simulink model "sampleModel1434"  (R2023a)
settings: Solver=VariableStepAuto  StartTime=0.0  StopTime=10.0  RelTol=1e-3
libraries: hdlsllib x3, simulink x1
settings Model: Creator=user1  LastModifiedBy=user1

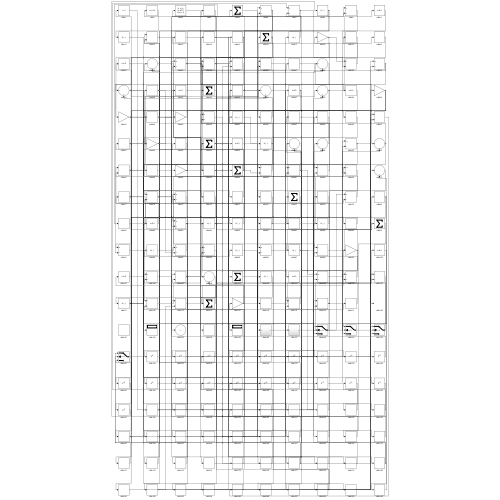
[thumbnail: Simulink's stored preview of the top-level diagram]
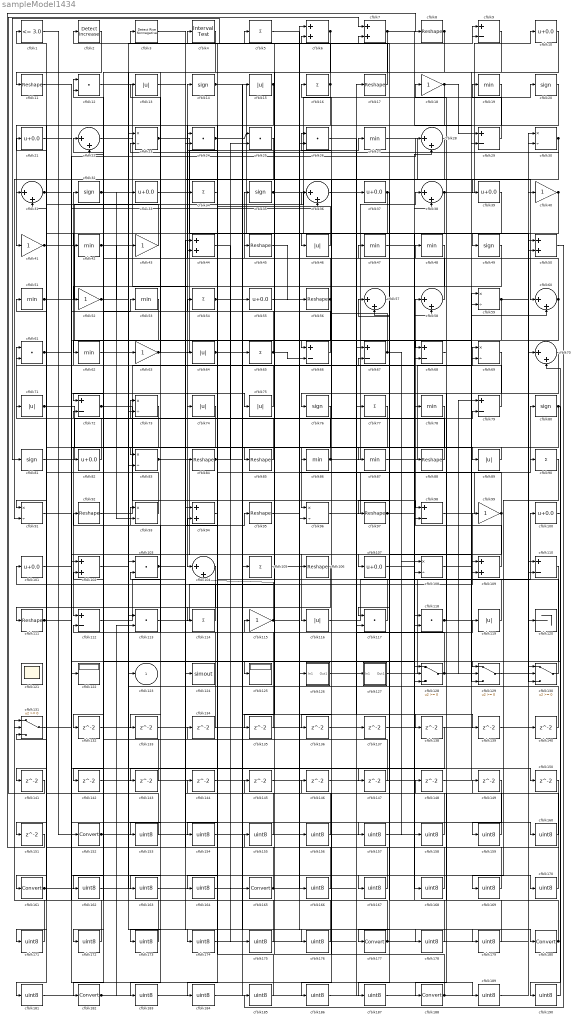
== system sampleModel1434 ==
  cfblk1 : hdlsllib/Logic and Bit Operations/Compare To Constant  relop=<=  const=3.0  OutDataTypeStr=boolean
  cfblk{10,21,33,37,39,55,82,100..101,107} (10 alike) : Bias  Bias=0.0  SaturateOnIntegerOverflow=off
  cfblk{6..7,44,50,94,102,109} (7 alike) : Sum
  cfblk{12,24..26,61,103,113,117..118} (9 alike) : DotProduct  OutDataTypeStr=Inherit: Inherit via internal rule
  cfblk{22,28,31,36,38,57..58,60,70,104} (10 alike) : Sum  Inputs=|++
  cfblk{5,16,34,54,65,77,90,105,114} (9 alike) : Sum  Inputs=+
  cfblk{8,11,17,45,56,84..85,88,92,95,97,106,111} (13 alike) : Reshape
  cfblk{23,30,59,69,73,83,91,93,96,108} (10 alike) : Product  Inputs=*/  RndMeth=Zero  SaturateOnIntegerOverflow=on
  cfblk{9,29,66..68,72,79,98,110,112} (10 alike) : Sum  Inputs=+-
  cfblk{18,40..41,43,52,63,99,115} (8 alike) : Gain
  cfblk{13,15,46,64,71,74..75,89,116,119} (10 alike) : Abs  SaturateOnIntegerOverflow=off
  cfblk120 : Terminator
  cfblk121 : Scope
      settings: Floating=on
  cfblk122 : Display
  cfblk124 : ToWorkspace  VariableName=simout  SaveFormat=Timeseries  SampleTime=-1
  cfblk125 : Display
  cfblk126 : Subsystem
      settings: LibrarySourceBlock=|
      | hdlsllib/Ports &
      | Subsystems/Subsystem
  cfblk127 : Subsystem
      settings: LibrarySourceBlock=|
      | hdlsllib/Ports &
      | Subsystems/Subsystem
  cfblk{128..131} (4 alike) : Switch  SaturateOnIntegerOverflow=off  InputSameDT=off
  cfblk{132..151} (20 alike) : Delay  SampleTime=1
  cfblk{14,20,32,35,49,76,80..81} (8 alike) : Signum
  cfblk{152,161,165,177,180,182,188} (7 alike) : DataTypeConversion  SaturateOnIntegerOverflow=off  RndMeth=Floor
  cfblk{153..160,162..164,166..176,178..179,181,183..187,189..190} (32 alike) : DataTypeConversion  OutDataTypeStr=uint8  SaturateOnIntegerOverflow=off  RndMeth=Floor
  cfblk{19,27,42,47..48,51,53,62,78,86..87} (11 alike) : MinMax
  cfblk2 : simulink/Logic and Bit Operations/Detect Increase  vinit=0.0  OutDataTypeStr=boolean
      settings: LibrarySourceBlock=|
      | hdlsllib/Logic and Bit
      | Operations/Detect
      | Increase
  cfblk3 : hdlsllib/Logic and Bit Operations/Detect Rise Nonnegative  vinit=0  OutDataTypeStr=boolean
  cfblk4 : hdlsllib/Logic and Bit Operations/Interval Test  IntervalClosedRight=on  uplimit=0.5  IntervalClosedLeft=on  lowlimit=-0.5  OutDataTypeStr=boolean
  cfblk123 : Outport  VectorParamsAs1DForOutWhenUnconnected=off
  wires:
  cfblk109/1 -> cfblk58/1
  cfblk74/1 -> cfblk112/1
  cfblk54/1 -> cfblk36/1, cfblk138/1, cfblk178/1
  cfblk86/1 -> cfblk38/1, cfblk31/2
  cfblk45/1 -> cfblk56/1
  cfblk27/1 -> cfblk60/1
  cfblk58/1 -> cfblk14/1
  cfblk117/1 -> cfblk3/1
  cfblk17/1 -> cfblk81/1
  cfblk46/1 -> cfblk4/1
  cfblk84/1 -> cfblk25/2, cfblk167/1, cfblk175/1
  cfblk33/1 -> cfblk104/1
  cfblk63/1 -> cfblk27/1, cfblk13/1
  cfblk127/1(Out1) -> cfblk100/1
  cfblk83/1 -> cfblk116/1, cfblk143/1
  cfblk103/1 -> cfblk68/2, cfblk176/1
  cfblk40/1 -> cfblk108/2, cfblk141/1, cfblk142/1
  cfblk100/1 -> cfblk129/1
  cfblk111/1 -> cfblk53/1, cfblk36/2, cfblk28/1
  cfblk79/1 -> cfblk32/1
  cfblk119/1 -> cfblk7/2
  cfblk129/1 -> cfblk130/2
  cfblk77/1 -> cfblk161/1
  cfblk44/1 -> cfblk165/1
  cfblk51/1 -> cfblk20/1, cfblk147/1
  cfblk37/1 -> cfblk76/1, cfblk97/1
  cfblk89/1 -> cfblk87/1
  cfblk78/1 -> cfblk111/1
  cfblk23/1 -> cfblk46/1, cfblk65/1
  cfblk66/1 -> cfblk22/1
  cfblk112/1 -> cfblk95/1
  cfblk118/1 -> cfblk129/2, cfblk18/1
  cfblk62/1 -> cfblk9/1
  cfblk16/1 -> cfblk41/1, cfblk2/1, cfblk31/1
  cfblk73/1 -> cfblk91/1
  cfblk88/1 -> cfblk26/1
  cfblk20/1 -> cfblk34/1
  cfblk68/1 -> cfblk48/1
  cfblk60/1 -> cfblk62/1, cfblk22/2
  cfblk72/1 -> cfblk98/1, cfblk79/2
  cfblk92/1 -> cfblk17/1
  cfblk14/1 -> cfblk49/1, cfblk128/3
  cfblk115/1 -> cfblk104/2, cfblk101/1, cfblk90/1
  cfblk56/1 -> cfblk35/1, cfblk83/2
  cfblk85/1 -> cfblk73/1
  cfblk38/1 -> cfblk10/1, cfblk173/1
  cfblk71/1 -> cfblk89/1, cfblk189/1
  cfblk87/1 -> cfblk69/1
  cfblk107/1 -> cfblk78/1
  cfblk70/1 -> cfblk188/1
  cfblk25/1 -> cfblk91/2
  cfblk128/1 -> cfblk59/2, cfblk79/1, cfblk12/2
  cfblk130/1 -> cfblk92/1
  cfblk6/1 -> cfblk85/1, cfblk183/1
  cfblk101/1 -> cfblk107/1
  cfblk59/1 -> cfblk130/3, cfblk118/2
  cfblk28/1 -> cfblk66/1
  cfblk29/1 -> cfblk19/1
  cfblk32/1 -> cfblk64/1, cfblk93/2
  cfblk30/1 -> cfblk23/2, cfblk132/1
  cfblk7/1 -> cfblk72/1, cfblk29/2
  cfblk12/1 -> cfblk84/1
  cfblk98/1 -> cfblk80/1
  cfblk10/1 -> cfblk129/3
  cfblk26/1 -> cfblk69/2
  cfblk8/1 -> cfblk24/2, cfblk162/1
  cfblk64/1 -> cfblk15/1, cfblk179/1
  cfblk41/1 -> cfblk126/1(In1), cfblk160/1
  cfblk80/1 -> cfblk96/1, cfblk190/1
  cfblk13/1 -> cfblk39/1
  cfblk42/1 -> cfblk123/1, cfblk6/2
  cfblk31/1 -> cfblk83/1, cfblk75/1
  cfblk2/1 -> cfblk11/1
  cfblk113/1 -> cfblk99/1
  cfblk105/1 -> cfblk180/1
  cfblk49/1 -> cfblk52/1
  cfblk110/1 -> cfblk182/1
  cfblk116/1 -> cfblk40/1
  cfblk82/1 -> cfblk61/1
  cfblk35/1 -> cfblk120/1, cfblk9/2
  cfblk114/1 -> cfblk93/1
  cfblk97/1 -> cfblk88/1, cfblk108/1
  cfblk34/1 -> cfblk114/1
  cfblk43/1 -> cfblk21/1
  cfblk19/1 -> cfblk42/1
  cfblk57/1 -> cfblk177/1
  cfblk93/1 -> cfblk71/1
  cfblk91/1 -> cfblk122/1
  cfblk3/1 -> cfblk86/1
  cfblk99/1 -> cfblk54/1, cfblk117/1, cfblk187/1
  cfblk22/1 -> cfblk124/1
  cfblk65/1 -> cfblk24/1, cfblk12/1, cfblk66/2
  cfblk52/1 -> cfblk128/2, cfblk43/1
  cfblk24/1 -> cfblk25/1, cfblk109/2
  cfblk4/1 -> cfblk73/2
  cfblk75/1 -> cfblk61/2
  cfblk108/1 -> cfblk60/2
  cfblk1/1 -> cfblk152/1
  cfblk21/1 -> cfblk125/1
  cfblk126/1(Out1) -> cfblk119/1
  cfblk18/1 -> cfblk29/1, cfblk164/1
  cfblk61/1 -> cfblk74/1, cfblk68/1
  cfblk81/1 -> cfblk33/1
  cfblk15/1 -> cfblk181/1, cfblk184/1
  cfblk96/1 -> cfblk30/2
  cfblk67/1 -> cfblk16/1, cfblk158/1
  cfblk132/1 -> cfblk98/2
  cfblk76/1 -> cfblk133/1
  cfblk133/1 -> cfblk130/1
  cfblk134/1 -> cfblk103/2
  cfblk9/1 -> cfblk135/1
  cfblk135/1 -> cfblk23/1
  cfblk48/1 -> cfblk136/1
  cfblk136/1 -> cfblk59/1
  cfblk137/1 -> cfblk128/1
  cfblk36/1 -> cfblk139/1
  cfblk139/1 -> cfblk30/1
  cfblk140/1 -> cfblk113/1
  cfblk141/1 -> cfblk7/1
  cfblk142/1 -> cfblk6/1
  cfblk143/1 -> cfblk72/2
  cfblk144/1 -> cfblk96/2
  cfblk145/1 -> cfblk58/2
  cfblk146/1 -> cfblk117/2
  cfblk147/1 -> cfblk112/2
  cfblk148/1 -> cfblk109/1
  cfblk11/1 -> cfblk150/1
  cfblk39/1 -> cfblk151/1
  cfblk151/1 -> cfblk8/1
  cfblk152/1 -> cfblk28/2, cfblk55/1
  cfblk138/1 -> cfblk153/1
  cfblk153/1 -> cfblk1/1
  cfblk94/1 -> cfblk154/1
  cfblk154/1 -> cfblk67/1
  cfblk150/1 -> cfblk155/1
  cfblk155/1 -> cfblk94/1
  cfblk55/1 -> cfblk156/1
  cfblk156/1 -> cfblk94/2
  cfblk5/1 -> cfblk157/1
  cfblk157/1 -> cfblk38/2
  cfblk158/1 -> cfblk5/1
  cfblk149/1 -> cfblk159/1
  cfblk159/1 -> cfblk67/2
  cfblk160/1 -> cfblk149/1
  cfblk161/1 -> cfblk82/1, cfblk63/1
  cfblk162/1 -> cfblk77/1
  cfblk106/1 -> cfblk163/1
  cfblk163/1 -> cfblk26/2
  cfblk164/1 -> cfblk106/1
  cfblk165/1 -> cfblk51/1, cfblk127/1(In1)
  cfblk95/1 -> cfblk166/1
  cfblk166/1 -> cfblk44/1
  cfblk167/1 -> cfblk44/2
  cfblk47/1 -> cfblk168/1
  cfblk168/1 -> cfblk145/1
  cfblk90/1 -> cfblk169/1
  cfblk169/1 -> cfblk47/1
  cfblk131/1 -> cfblk170/1
  cfblk170/1 -> cfblk103/1
  cfblk104/1 -> cfblk171/1
  cfblk171/1 -> cfblk131/1
  cfblk53/1 -> cfblk172/1
  cfblk172/1 -> cfblk131/2
  cfblk173/1 -> cfblk131/3
  cfblk102/1 -> cfblk174/1
  cfblk174/1 -> cfblk37/1
  cfblk175/1 -> cfblk102/1
  cfblk176/1 -> cfblk102/2
  cfblk177/1 -> cfblk144/1, cfblk140/1, cfblk45/1
  cfblk178/1 -> cfblk57/1
  cfblk179/1 -> cfblk57/2
  cfblk180/1 -> cfblk148/1, cfblk118/1
  cfblk181/1 -> cfblk105/1
  cfblk182/1 -> cfblk137/1, cfblk113/2
  cfblk183/1 -> cfblk110/1
  cfblk184/1 -> cfblk110/2
  cfblk50/1 -> cfblk185/1
  cfblk185/1 -> cfblk134/1
  cfblk69/1 -> cfblk186/1
  cfblk186/1 -> cfblk50/1
  cfblk187/1 -> cfblk50/2
  cfblk188/1 -> cfblk146/1, cfblk115/1
  cfblk189/1 -> cfblk70/1
  cfblk190/1 -> cfblk70/2

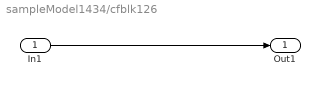
== system sampleModel1434/cfblk126 ==
  In1 : Inport
  Out1 : Outport
  wires:
  In1/1 -> Out1/1

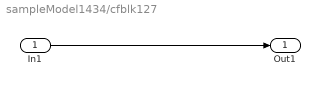
== system sampleModel1434/cfblk127 ==
  In1 : Inport
  Out1 : Outport
  wires:
  In1/1 -> Out1/1
